simulink model "ImuCalibrator"  (R2018a)
settings: Solver=FixedStepDiscrete  StartTime=0.0  StopTime=inf  FixedStep=1/Fss  RelTol=1e-3
PreLoadFcn:
  | modelDef = getModelDef();
  | Fss = 1;  % nominal IMU sampling rate
  | 
  | gyroCalBiases = [0;0;0];
  | gyroCalMatrix = eye(3);
  | gyroGsensMatrix = zeros(3,3);
  | 
  | accelCalBiases = [0;0;0];
  | accelCalMatrix = eye(3);
  | 
  | imuPar = getImuPar('lmvpUncalibrated');
  | 
  | lastUsedMgyr = zeros(3,3);
undefined symbols (not defined in the file or in its folder): numStates
libraries: simulink x5, vrlib x5, dspinverses x4, dspsigops x2, dspindex x2, dspstat3 x1, simulink_extras x1, dspmtrx3 x1, dspsnks4 x1, dspsrcs4 x1, dspswit3 x1
(part 2 of 2)

== matlab function ImuCalibrator/AINS/time update/MATLAB Function ==
  data: omega input; Q output size=[modelDef.numStates, modelDef.numStates]; f_ib input; Dt input; Cbn input; modelDef parameter; imuPar parameter
function Q  = calculate_Q(omega, f_ib, Dt, Cbn, modelDef, imuPar)

% order of the states:
% 1:3   phi
% 4:6   dw
% 7:9   dr
% 10:12 dv
% 13:15 df  (if modelDef.trackAccelBiases)
% 16:24 dM_gyro in column-major order (if modelDef.trackGyroSfma)
% 25:33 dM_accel in column-major order (if modelDef.trackAccelSfma)

Q = zeros(modelDef.numStates, modelDef.numStates);

omega = reshape(omega,3,1); 
f_ib = reshape(f_ib, 3,1);

Qphi = diag((imuPar.gyroArwRadPerRtSec^2)*[Dt Dt Dt]);  
Qdw = diag((imuPar.gyroBrwRadPerSecPerRtSec^2)*[Dt Dt Dt]);
Qdv = diag((imuPar.accelVrwMetersPerSecPerRtSec^2)*[Dt Dt Dt]);
Qdf = diag((imuPar.accelBrwMetersPerSec2PerRtSec^2)*[Dt Dt Dt]);


%bump up Q for unmodelled states
if ~modelDef.trackGyroSfma % gyro scale factor and misalignment not tracked
   gyroSfSigmaBod = imuPar.gyroScaleUncert*omega;
   gyroMaSigmaBod = imuPar.gyroAlignUncert*sqrt(omega'*omega*[1 1 1]-omega'.*omega');   
   QgyroMa = Cbn*diag(gyroMaSigmaBod.^2)*Cbn'*Dt; 
   QgyroSf = Cbn*diag(gyroSfSigmaBod.^2)*Cbn'*Dt; 
   Qphi = Qphi + QgyroMa + QgyroSf;   
end

if ~modelDef.trackGyroGsens %  gyro g sensitivity not tracked 
   gGsensSigmaBod = imuPar.gyroGsensUncert*sqrt(f_ib'*f_ib*[1 1 1]-f_ib'.*f_ib');   
   QgGsens = Cbn*diag(gGsensSigmaBod.^2)*Cbn'*Dt; 
   Qphi = Qphi + QgGsens;   
end

if ~modelDef.trackAccelSfma  % accel scale factor and misalignment not tracked
   accelSfSigmaBod = imuPar.accelScaleUncert*f_ib;
   accelMaSigmaBod = imuPar.accelAlignUncert*sqrt(f_ib'*f_ib*[1 1 1]-f_ib'.*f_ib');   
   QaccelMa = Cbn*diag(accelMaSigmaBod.^2)*Cbn'*Dt; 
   QaccelSf = Cbn*diag(accelSfSigmaBod.^2)*Cbn'*Dt; 
   Qdv = Qdv + QaccelMa + QaccelSf;   
end

Q(1:3, 1:3) = Qphi;
Q(4:6, 4:6) = Qdw;
Q(10:12, 10:12) = Qdv;
Q(13:15, 13:15) = Qdf;

== matlab function ImuCalibrator/AINS/time update/MATLAB Function1 ==
  data: imuPar output Bus: imuPar
function imuPar = imuPar

imuPar.gyroArwDegPerRtHr = 0.25;
imuPar.gyroArwRadPerRtSec = imuPar.gyroArwDegPerRtHr * pi/180/60;
imuPar.gyroBrwDegPerHrPerRtHr = 0;
imuPar.gyroBrwRadPerSecPerRtSec = imuPar.gyroBrwDegPerHrPerRtHr * pi/180/3600/60;
imuPar.gyroScaleUncertainty = 0.001;
imuPar.gyroAlignUncertainty = 0.01;
imuPar.gyroGsensUncertainty = 0.001;

== matlab function ImuCalibrator/AINS/time update/MATLAB Function2 ==
  settings: updateMethod=DISCRETE  sampleTime=inf
  data: modelDef output Bus: modelDef; numStates input
function modelDef = modelDef(numStates)

modelDef.trackAccelBiases = true;
modelDef.trackAccelSfma = true;
modelDef.trackGyroSfma = true;
modelDef.trackGyroGsens = false;

modelDef.numStates = numStates;

== matlab function ImuCalibrator/AINS/time update/MATLAB Function3 ==
  data: omega input; Phi output size=[modelDef.numStates, modelDef.numStates]; fbod input; Dt input; Cbn input; modelDef parameter
function Phi  = calculate_Phi(omega, fbod, Dt, Cbn, modelDef)

% order of the states:
% 1:3   phi
% 4:6   dw
% 7:9   dr
% 10:12 dv
% 13:15 df  (if modelDef.trackAccelBiases)
% 16:24 dM_gyro in column-major order (if modelDef.trackGyroSfma)
% 25:33 dM_accel in column-major order (if modelDef.trackAccelSfma)
% 34:42 dG_gyro in column-major order (if modelDef.trackGyroGsens)

Phi = eye(modelDef.numStates);

DtC = Dt*Cbn;

Phi(1:3,4:6) = -DtC;  % propagate dw to phi
Phi(7:9, 10:12) = Dt*eye(3);  % propagate dv to dr
Phi(10:12, 1:3) = Dt*skew(Cbn*fbod);  % propagate phi to dv

if modelDef.trackAccelBiases
    Phi(10:12, 13:15) = DtC;   % propagate df to dv
end

if modelDef.trackGyroSfma  % propagate dM_gyro to phi
    Phi(1:3, 16:18) = -DtC*omega(1);
    Phi(1:3, 19:21) = -DtC*omega(2);
    Phi(1:3, 22:24) = -DtC*omega(3);
end

if modelDef.trackAccelSfma  % propagate dM_accel to dv
    Phi(10:12, 25:27) = DtC*fbod(1);
    Phi(10:12, 28:30) = DtC*fbod(2);
    Phi(10:12, 31:33) = DtC*fbod(3);
end

if modelDef.trackGyroGsens  % propagate dG_gyro to phi
    Phi(1:3, 34:36) = -DtC*fbod(1);
    Phi(1:3, 37:39) = -DtC*fbod(2);
    Phi(1:3, 40:42) = -DtC*fbod(3);
end


function res=skew(inp_vr)
res=[0 			-inp_vr(3)	inp_vr(2); ...
     inp_vr(3)	0			-inp_vr(1);...
	 -inp_vr(2)	inp_vr(1)	0];

== matlab function ImuCalibrator/AINS/zero velocity update/MATLAB Function1 ==
  data: S output; P input; K output; H input; R input
function [S,K] = calcKalmanGain(P, H, R)

PHT = P*H';
S = H*PHT + R;
K = PHT/S;

== matlab function ImuCalibrator/readFromFile/printTime/MATLAB Function ==
  data: u input
function  printTime(u)
%#codegen

% using fileId = 1  only generates a printf in the generated code
% fileId = 2 also causes prints in the matlab console

fprintf(1, "\r %f", u);

== matlab function ImuCalibrator/AINS/initialize states and covariances/set P/MATLAB Function1 ==
  data: initialRotUncert input; initialPosUncert input; initialVelUncert input; P0 output size=[modelDef.numStates, modelDef.numStates]; modelDef parameter; imuPar parameter
function P0  = calculate_P0(initialRotUncert, initialPosUncert, initialVelUncert, modelDef, imuPar)

% order of the states:
% 1:3   phi
% 4:6   dw
% 7:9   dr
% 10:12 dv
% 13:15 df  (if modelDef.trackAccelBiases)
% 16:24 dM_gyro in column-major order (if modelDef.trackGyroSfma)
% 25:33 dM_accel in column-major order (if modelDef.trackAccelSfma)
% 34:42 dG_gyro in column-major order (if modelDef.trackGyroGsens)

P0 = zeros(modelDef.numStates, modelDef.numStates);

P0(1:3, 1:3) = diag(initialRotUncert.^2);
P0(4:6, 4:6) = eye(3)*(imuPar.gyroBiasUncert.^2);
P0(7:9, 7:9) = diag(initialPosUncert.^2);
P0(10:12, 10:12) = diag(initialVelUncert.^2);


if modelDef.trackAccelBiases
    P0(13:15, 13:15) = eye(3)*(imuPar.accelBiasUncert.^2);
end

if modelDef.trackGyroSfma  
    vec9 = ones(9,1)*imuPar.gyroAlignUncert^2;
    vec9([1 5 9]) = imuPar.gyroScaleUncert^2;
    P0(16:24, 16:24) = diag(vec9);
end

if modelDef.trackAccelSfma  % propagate dM_accel to dv
    vec9 = ones(9,1)*imuPar.accelAlignUncert^2;
    vec9([1 5 9]) = imuPar.accelScaleUncert^2;
    if modelDef.accelDefinesExtrinsics
        vec9([4 7]) = 0.0001^2; % x accel has no misalignment so picks up no component of y or z accelerations
        vec9(8) = 0.0001^2;  % y accel has no tilt out of xy plane, so picks up no component of z acceleration
    end
    P0(25:33, 25:33) = diag(vec9);
end

if modelDef.trackGyroGsens
    vec9 = ones(9,1)*imuPar.gyroGsensUncert^2;
    P0(34:42, 34:42) = diag(vec9);
end

== matlab function ImuCalibrator/AINS/gravity meas update/MATLAB Function3 ==
  data: P input; Pplus output; K input; H input; R input; IminKH output
function [Pplus, IminKH] = josephCovarianceUpdate(P, K, H, R)

IminKH = eye(size(P)) - K*H;
Pplus = IminKH*P*IminKH' + K*R*K';

== matlab function ImuCalibrator/AINS/zero velocity update/MATLAB Function3 ==
  data: P input; Pplus output; K input; H input; R input; IminKH output
function [Pplus, IminKH] = josephCovarianceUpdate(P, K, H, R)

IminKH = eye(size(P)) - K*H;
Pplus = IminKH*P*IminKH' + K*R*K';

== matlab function ImuCalibrator/AINS/zero velocity update/update the underlying states/MATLAB Function ==
  data: inp_vr input; res output
function res=skew(inp_vr)
res=[0 			-inp_vr(3)	inp_vr(2); ...
     inp_vr(3)	0			-inp_vr(1);...
	 -inp_vr(2)	inp_vr(1)	0];

== matlab function ImuCalibrator/AINS/report output/MATLAB Function1 ==
  data: Cbn input; quat output size=[4,1]
function quat=dcm2quat(Cbn)

%dcm (Cba) to quaternion (qba)
%Cba:B to A transformation matrix
%qba:B to A quaternion

%Implementation of savage(3-47)


tr=Cbn(1,1)+Cbn(2,2)+Cbn(3,3);
Pa=1+tr;
Pb=1+2*Cbn(1,1)-tr;
Pc=1+2*Cbn(2,2)-tr;
Pd=1+2*Cbn(3,3)-tr;

quat=zeros(4,1);
if (Pa>=Pb && Pa>=Pc && Pa>=Pd)
    quat(1)=0.5*sqrt(Pa);
    quat(2)=(Cbn(3,2)-Cbn(2,3))/4/quat(1);
    quat(3)=(Cbn(1,3)-Cbn(3,1))/4/quat(1);
    quat(4)=(Cbn(2,1)-Cbn(1,2))/4/quat(1);
elseif (Pb>=Pc && Pb>=Pd)
    quat(2)=0.5*sqrt(Pb);
    quat(3)=(Cbn(2,1)+Cbn(1,2))/4/quat(2);
    quat(4)=(Cbn(1,3)+Cbn(3,1))/4/quat(2);
    quat(1)=(Cbn(3,2)-Cbn(2,3))/4/quat(2);
elseif (Pc>=Pd)
    quat(3)=0.5*sqrt(Pc);
    quat(4)=(Cbn(3,2)+Cbn(2,3))/4/quat(3);
    quat(1)=(Cbn(1,3)-Cbn(3,1))/4/quat(3);
    quat(2)=(Cbn(2,1)+Cbn(1,2))/4/quat(3);
else
    quat(4)=0.5*sqrt(Pd);
    quat(1)=(Cbn(2,1)-Cbn(1,2))/4/quat(4);
    quat(2)=(Cbn(1,3)+Cbn(3,1))/4/quat(4);
    quat(3)=(Cbn(3,2)+Cbn(2,3))/4/quat(4);
end

if (quat(1)<=0)
    quat=-quat;
end

== matlab function ImuCalibrator/Atomic Subsystem/MATLAB Function ==
  data: values input; closeFile input
function asciiWriteLine(values, closeFile)

persistent fid

if isempty(fid)
    fid = fopen('GyroAccelDt.txt', 'w'); %open for writing, discard current contents it it already exists
end


for i=1:length(values)
    fprintf(fid, " %9.7f", values(i) );
end
fprintf(fid, "\n");

if closeFile
    fclose(fid);
end

== matlab function ImuCalibrator/readFromFile/MATLAB Function1 ==
  data: datarow output; EOF output
function [datarow, EOF] = readLineAscii()

persistent data data2 nrows row

if isempty(data)
    % row format = # SeqID, DeviceID, timestamp (sec), gyroXYZ (rad/sec), accelXYZ (m/s^2), temperature (degC)
    coder.varsize('data', [500000, 10], [1 0]);  % ten columns,  up to 200k rows
    data = load('imudata.txt', '-ascii'); 
    
    validTimestamp = data(:,3) > 0.001;
    data2 = data(validTimestamp, [4 5 6 7 8 9 3]); % select just the useful columns and rows
    nrows = size(data2, 1);
    row = 2;  % skip the first row since we need delta-t's

end

datarow = data2(row,:)';
datarow(7) = data2(row,7) - data2(row-1,7); % calculate Delta-t

EOF = row >= nrows;
row = row + 1;

== matlab function ImuCalibrator/AINS/gravity meas update/MATLAB Function2 ==
  data: inp_vr input; res output
function res=skew(inp_vr)
res=[0 			-inp_vr(3)	inp_vr(2); ...
     inp_vr(3)	0			-inp_vr(1);...
	 -inp_vr(2)	inp_vr(1)	0];

== matlab function ImuCalibrator/AINS/compass meas update/MATLAB Function1 ==
  data: S output; P input; K output; H input; R input
function [S,K] = calcKalmanGain(P, H, R)

PHT = P*H';
S = H*PHT + R;
K = PHT/S;

== matlab function ImuCalibrator/AINS/compass meas update/MATLAB Function3 ==
  data: P input; Pplus output; K input; H input; R input; IminKH output
function [Pplus, IminKH] = josephCovarianceUpdate(P, K, H, R)

IminKH = eye(size(P)) - K*H;
Pplus = IminKH*P*IminKH' + K*R*K';

== matlab function ImuCalibrator/AINS/compass meas update/update the Cbn with the errors/MATLAB Function ==
  data: inp_vr input; res output
function res=skew(inp_vr)
res=[0 			-inp_vr(3)	inp_vr(2); ...
     inp_vr(3)	0			-inp_vr(1);...
	 -inp_vr(2)	inp_vr(1)	0];
